simulink model "EqRealNiMH"  (R2015a)
settings: configuration reference "SIMULATION_CONFIGURATION" (kept outside this file)
settings Model: CovSFcnEnable=off  Creator=moritz  LastModifiedBy=moritz
settings ConfigSetRef: SourceLocation=Base Workspace

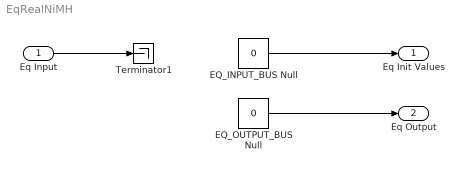
== system EqRealNiMH ==
  Eq Input : Inport  OutDataTypeStr=Bus: EQ_INPUT_BUS  BusOutputAsStruct=on
  EQ_INPUT_BUS Null : Constant  Value=0  OutDataTypeStr=Bus: EQ_INPUT_BUS  SampleTime=-1
  EQ_OUTPUT_BUS Null : Constant  Value=0  OutDataTypeStr=Bus: EQ_OUTPUT_BUS  SampleTime=-1
  Terminator1 : Terminator
  Eq Init Values : Outport  OutDataTypeStr=Bus: EQ_INPUT_BUS  BusOutputAsStruct=on
  Eq Output : Outport  Port=2  OutDataTypeStr=Bus: EQ_OUTPUT_BUS  BusOutputAsStruct=on
  wires:
  EQ_INPUT_BUS Null/1 -> Eq Init Values/1
  Eq Input/1 -> Terminator1/1
  EQ_OUTPUT_BUS Null/1 -> Eq Output/1
